simulink model "motion_example2"  (Simulink 10.0)
settings: Solver=ode45  StartTime=0.0  StopTime=3  RelTol=1e-3  EnableMultiTasking=on
undefined symbols (not defined in the file): Ac, Bc, Cc, Dc
libraries: motion x5, simulink3 x2
settings Model: Creator=bhisma  LastModifiedBy=bhisma  ExtModeTrigMode=oneshot  ExtModeArmWhenConnect=off
settings DataIOCC: SignalLoggingSaveFormat=ModelDataLogs
settings OptimizationCC: BooleanDataType=off  LifeSpan=auto
settings DebuggingCC: SaveWithParameterizedLinksMsg=none  SignalResolutionControl=TryResolveAllWithWarning  MultiTaskDSMMsg=warning  MultiTaskCondExecSysMsg=none  SFUnexpectedBacktrackingDiag=error  SFNoUnconditionalDefaultTransitionDiag=error  SFExecutionAtInitializationDiag=warning  ArithmeticOperatorsInVariantConditions=error
settings HardwareCC: ProdBitPerPointer=64  ProdBitPerSizeT=64  ProdBitPerPtrDiffT=64  ProdLargestAtomicFloat=Float  ProdIntDivRoundTo=Zero  ProdEndianess=LittleEndian  ProdWordSize=64  ProdHWDeviceType=Intel->x86-64 (Windows64)  TargetUnknown=on
settings SFSimCC: SimUseLocalCustomCode=on  CustomCodeUndefinedFunction=FilterOut
settings RTWCC: RTWUseLocalCustomCode=on
settings CodeAppCC: StateflowObjectComments=off
settings GRTTargetCC: TargetLangStandard=C99 (ISO)
settings ConfigComp: CovMetricSettings=dwe  CovSaveCumulativeToWorkspaceVar=off  CovSaveSingleToWorkspaceVar=off

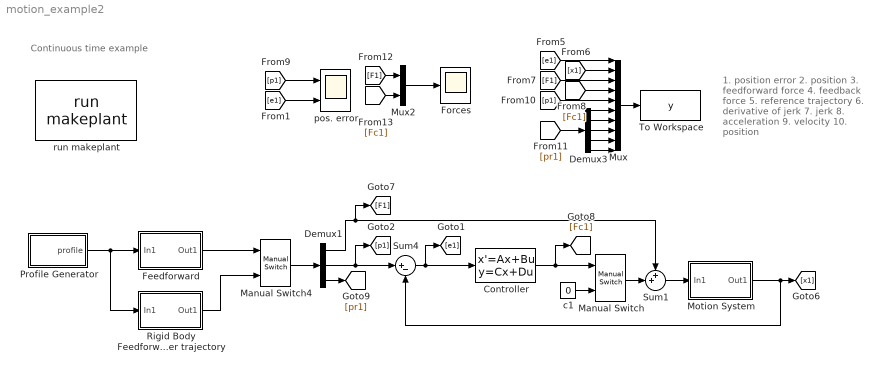
== system motion_example2 ==
  note: 1.   position error
      | 2.   position
      | 3.   feedforward force
      | 4.   feedback force
      | 5.   reference trajectory
      | 6.   derivative of jerk
      | 7.   jerk
      | 8.   acceleration
      | 9.   velocity
      | 10. position
  note: Continuous time example
  Controller : StateSpace  A=Ac  B=Bc  C=Cc  D=Dc  InitialCondition=0
  Demux1 : Demux  Outputs=[1 1 5]
  Demux3 : Demux  Outputs=5
  Feedforward : Subsystem  BlockChoice=4th order continuous
      link override 4th order cont: m1=30  m2=0  k1=20  k2=0  k12=0
      link override 4th order continuous: c=6e5
      settings: AttributesFormatString=%<BlockChoice>  TemplateBlock=motion/Feedforward Controllers/Feedforward  MemberBlocks=2nd order continuous,2nd order discrete,3d order continuous,3d order discrete,4th order continuous,4th order digital,4th order discrete
  Forces : Scope
  Manual Switch : simulink3/Nonlinear/Manual Switch  sw=1  action=0
      settings: SourceProductName=Simulink  SourceProductBaseCode=SL
  Manual Switch4 : simulink3/Nonlinear/Manual Switch  sw=1  action=0
      settings: SourceProductName=Simulink  SourceProductBaseCode=SL
  Motion System : Subsystem  BlockChoice=Parametrized 4th order
      link override Parametrized 4th order: k1=10  k2=10  c=6e5
      settings: AttributesFormatString=%<BlockChoice>  TemplateBlock=motion/Motion Systems1/Motion System  MemberBlocks=2nd order,4th order,6th order,Parametrized 4th order
  Mux : Mux  Inputs=10
  Mux2 : Mux  Inputs=2
  Profile Generator : Subsystem  BlockChoice=Derivative of Jerk
      link override Derivative of Jerk: Ts=0  j=45
      settings: AttributesFormatString=%<BlockChoice>  TemplateBlock=motion/Profile Generators/Profile Generator  MemberBlocks=Acceleration,Derivative of Jerk,Jerk,dJerk with error correction
  Rigid Body Feedforward with 4th order trajectory : Subsystem  BlockChoice=4th order continuous
      link override 4th order cont: k1=10  k2=10
      link override 4th order continuous: m1=30  m2=0  k1=20  k2=0  k12=0
      settings: AttributesFormatString=%<BlockChoice>  TemplateBlock=motion/Feedforward Controllers/Feedforward  MemberBlocks=2nd order continuous,2nd order discrete,3d order continuous,3d order discrete,4th order continuous,4th order digital,4th order discrete
  Sum1 : Sum  Inputs=++|  SaturateOnIntegerOverflow=on  InputSameDT=on  OutDataTypeStr=Inherit: Same as first input
  Sum4 : Sum  Inputs=|+-  SaturateOnIntegerOverflow=on  InputSameDT=on  OutDataTypeStr=Inherit: Same as first input
  To Workspace : ToWorkspace  VariableName=y  SaveFormat=Structure With Time  SampleTime=2e-4
  c1 : Constant  Value=0
  pos. error : Scope  NumInputPorts=2
  run makeplant : motion/General/run makeplant
  wires:
  Sum1/1 -> Motion System/1(In1)
  Sum4/1 -> [e1], Controller/1
  Mux/1 -> To Workspace/1
  Profile Generator/1(profile) -> Feedforward/1(In1), Rigid Body Feedforward with 4th order trajectory/1(In1)
  Motion System/1(Out1) -> [x1], Sum4/2
  Demux1/2 -> Sum4/1, [p1]
  Demux1/1 -> [F1], Sum1/1
  Mux2/1 -> Forces/1
  Demux3/1 -> Mux/6
  Demux3/2 -> Mux/7
  Demux3/3 -> Mux/8
  Demux3/4 -> Mux/9
  [e1] -> pos. error/2
  [p1] -> pos. error/1
  [e1] -> Mux/1
  [x1] -> Mux/2
  [F1] -> Mux/3
  [Fc1] -> Mux/4
  [p1] -> Mux/5
  Demux1/3 -> [pr1]
  [pr1] -> Demux3/1
  c1/1 -> Manual Switch/2
  Controller/1 -> [Fc1], Manual Switch/1
  Manual Switch/1 -> Sum1/2
  [F1] -> Mux2/1
  Feedforward/1(Out1) -> Manual Switch4/1
  Manual Switch4/1 -> Demux1/1
  Rigid Body Feedforward with 4th order trajectory/1(Out1) -> Manual Switch4/2
  [Fc1] -> Mux2/2
  Demux3/5 -> Mux/10

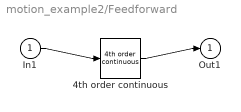
== system motion_example2/Feedforward ==
  In1 : Inport
  4th order continuous : motion/Feedforward Controllers/4th order continuous  m1=20  m2=10  k1=10  k2=10  c=6e5  k12=500
  Out1 : Outport
  wires:
  In1/1 -> 4th order continuous/1
  4th order continuous/1 -> Out1/1

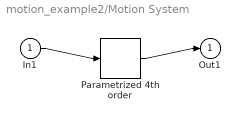
== system motion_example2/Motion System ==
  In1 : Inport
  Parametrized 4th order : motion/Motion Systems1/Parametrized 4th order  m1=20  m2=10  k1=10  k2=10  c=6e5  k12=500
  Out1 : Outport
  wires:
  In1/1 -> Parametrized 4th order/1
  Parametrized 4th order/1 -> Out1/1

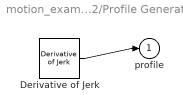
== system motion_example2/Profile Generator ==
  Derivative of Jerk : motion/Profile Generators/Derivative of Jerk  t0=.3  x=1  v=1  a=5  j=45  d=1000  Ts=0
  profile : Outport
  wires:
  Derivative of Jerk/1 -> profile/1

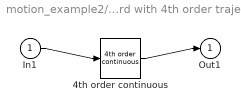
== system motion_example2/Rigid Body Feedforward with 4th order trajectory ==
  In1 : Inport
  4th order continuous : motion/Feedforward Controllers/4th order continuous  m1=30  m2=0  k1=20  k2=0  c=6e5  k12=0
  Out1 : Outport
  wires:
  In1/1 -> 4th order continuous/1
  4th order continuous/1 -> Out1/1
